simulink model "platoon_project_string_stability2"  (Simulink 8.9)
settings: Solver=VariableStepAuto  StartTime=0.0  StopTime=20  FixedStep=0.1  RelTol=1e-3  EnableMultiTasking=on
values from neighbouring files (symbols this model uses):
  k1 = 1.3244    [platoon_stability.m]    (also in platoon_stability_ed.m = 0.0244)
  k2 = -1.2211    [platoon_stability.m]    (also in platoon_stability_ed.m = -1.7211)
  q = 0.1    [platoon_stability.m]    (also in platoon_stability_ed.m = 0.2)
  tau = 1.34    [platoon_stability.m]    (also in platoon_stability_ed.m = 1.24)
  tnet_table = [57.5127074443 119.897368421 182.282029398 223.675296349 261.549751738 274.206057597 279.305263158 283.689473684 288.073684211 292.467532318 296.875779086 301.284025854 ... (400 elements, 20x20)]    [enginemap.mat]    (also in genmap.m = griddata(map_ford(:,1), map_ford(:,4), map_ford(:,2), we_tab)
  we_max = 471.2    [enginemap.mat]    (also in genmap.m = max(map_ford(:,1)))
  we_min = 57.6    [enginemap.mat]    (also in genmap.m = min(map_ford(:,1)))
undefined symbols (not defined in the file or in its folder): c_aero, delay_brake, F_roll, h, I_e, I_wheel, KB, mass, max_throttle, max_throttle_rate, min_throttle, mu_B, mu_C, mu_D, mu_E, P_po, Rdrive, sigbuilder_block, tau_brake, tau_throttle, throttle_o, w_wheel_o, we_o, x_dot_o
libraries: simulink x8
(part 2 of 3)

== system platoon_project_string_stability2/4th Vehicle/Engine Model ==
  note: engine map이 저장되어있다
      | 2-D Lookup table
      |
      | input : Throttle angle, Engine speed
      | output : Engine torque
  Tractive Force : Inport
  Throttle Angle : Inport  Port=2
  Brake Torque : Inport  Port=3
  Gear Ratio : Inport  Port=4
  1/(I_e+4*I_w*R^2) : Fcn  Expr=u(1)/(I_e+4*I_wheel*u(2)^2)
  Integrator : Integrator  InitialCondition=we_o  LimitOutput=on  UpperSaturationLimit=[we_max]  LowerSaturationLimit=[we_min]
  Mux : Mux  Inputs=2
  Product : Product  SaturateOnIntegerOverflow=on  RndMeth=Zero  InputSameDT=on  OutDataTypeStr=Inherit: Same as first input
  Sum : Sum  Inputs=+|-  SaturateOnIntegerOverflow=on  InputSameDT=on  OutDataTypeStr=Inherit: Same as first input
  Sum1 : Sum  SaturateOnIntegerOverflow=on  InputSameDT=on  OutDataTypeStr=Inherit: Same as first input
  T_net : Lookup2D  RowIndex=alpha_table  ColumnIndex=we_table  Table=tnet_table  SaturateOnIntegerOverflow=on  InputSameDT=on
  wheel radius : Gain  Gain=h  Multiplication=Matrix(K*u)  SaturateOnIntegerOverflow=on  OutDataTypeStr=Inherit: Same as input  ParamDataTypeStr=Inherit: Same as input
  Engine Speed : Outport
  Engine Torque : Outport  Port=2
  wires:
  Throttle Angle/1 -> T_net/1
  Integrator/1 -> Engine Speed/1, T_net/2  "w"
  1/(I_e+4*I_w*R^2)/1 -> Integrator/1  "w_dot"
  Tractive Force/1 -> wheel radius/1
  wheel radius/1 -> Sum1/1
  Brake Torque/1 -> Sum1/2
  Product/1 -> Sum/2
  Sum1/1 -> Product/1
  Gear Ratio/1 -> Product/2, Mux/2
  Sum/1 -> Mux/1
  Mux/1 -> 1/(I_e+4*I_w*R^2)/1
  T_net/1 -> Engine Torque/1, Sum/1

== system platoon_project_string_stability2/4th Vehicle/Gear Shift ==
  note: [1 1 1]인 [n,1] 행렬과
      | 반환행렬을 곱해서
      | 스칼라값(기어값)을 만든다
  note: 현재 차량 속도 vs 기어변속 속도를 비교한다
      | [0; 1; 1] 같은 [1,n]행렬이 반환된다
  Vehicle Speed : Inport
  Convert m/s to mph : Gain  Gain=3.6/1.6  SaturateOnIntegerOverflow=on  OutDataTypeStr=Inherit: Same as input  ParamDataTypeStr=Inherit: Same as input
  Direct Look-Up of Gear ratio : LookupNDDirect  NumberOfTableDimensions=1  Table=[0.3423,0.6378,1.0,1.4184]
  Get gear-1 : Gain  Gain=ones(1,3)  Multiplication=Matrix(K*u)  SaturateOnIntegerOverflow=on  OutDataTypeStr=Inherit: Same as input  ParamDataTypeStr=Inherit: Same as input
  Relational Operator : RelationalOperator  Operator=>  RndMeth=Nearest  InputSameDT=on
  Shift Speeds : Constant  Value=[15 32 67]
  Gear Ratio : Outport
  wires:
  Shift Speeds/1 -> Relational Operator/2
  Relational Operator/1 -> Get gear-1/1
  Convert m/s to mph/1 -> Relational Operator/1
  Get gear-1/1 -> Direct Look-Up of Gear ratio/1
  Vehicle Speed/1 -> Convert m/s to mph/1
  Direct Look-Up of Gear ratio/1 -> Gear Ratio/1

== system platoon_project_string_stability2/4th Vehicle/Throttle Actuator ==
  Command : Inport
  Integrator : Integrator  InitialCondition=throttle_o  LimitOutput=on  UpperSaturationLimit=max_throttle  LowerSaturationLimit=min_throttle
  Saturation : Saturate  UpperLimit=max_throttle_rate  LowerLimit=-max_throttle_rate
  Sum : Sum  Inputs=-+|  SaturateOnIntegerOverflow=on  InputSameDT=on  OutDataTypeStr=Inherit: Same as first input
  Throttle Time Constant : Gain  Gain=1/tau_throttle  SaturateOnIntegerOverflow=on  OutDataTypeStr=Inherit: Same as input  ParamDataTypeStr=Inherit: Same as input
  Angle : Outport
  wires:
  Command/1 -> Sum/2
  Integrator/1 -> Angle/1, Sum/1
  Sum/1 -> Throttle Time Constant/1
  Throttle Time Constant/1 -> Saturation/1
  Saturation/1 -> Integrator/1

== system platoon_project_string_stability2/4th Vehicle/Vehicle Dynamics ==
  note: 타이어저항 F_road
  note: v
  note: v_dot
  note: 공기저항 F_air
  note: 구름저항 F_roll
  note: Initial Velocity = 21 [m/s]
  Tractive Force : Inport
  Aerodynamic Drag : Fcn  Expr=c_aero*u^2
  Divide by Mass : Gain  Gain=1/mass  Multiplication=Matrix(K*u)  SaturateOnIntegerOverflow=on  OutDataTypeStr=Inherit: Same as input  ParamDataTypeStr=Inherit: Same as input
  Integrator : Integrator  InitialCondition=x_dot_o  LimitOutput=on  LowerSaturationLimit=0
  Rolling Resistance : Constant  Value=F_roll
  Sum1 : Sum  Inputs=--+  SaturateOnIntegerOverflow=on  InputSameDT=on  OutDataTypeStr=Inherit: Same as first input
  Velocity : Outport
  Acceleration : Outport  Port=2
  wires:
  Tractive Force/1 -> Sum1/3
  Divide by Mass/1 -> Acceleration/1, Integrator/1
  Integrator/1 -> Velocity/1, Aerodynamic Drag/1
  Sum1/1 -> Divide by Mass/1
  Rolling Resistance/1 -> Sum1/2
  Aerodynamic Drag/1 -> Sum1/1

== system platoon_project_string_stability2/4th Vehicle/Wheel Dynamics ==
  note: 여기 주석!
  note: Tractive Force는 4바퀴 전부 더한다
  note: 평균을 계산해서 하나의 Wheel Speed를 만든다
  note: 브레이크는 전체 유압을
      | 전륜, 후륜에 특정비율로 분배한다
      | 40% (전륜), 60% (후륜)
  Vehicle Speed : Inport
  T_shaft : Inport  Port=2
  Brake Torque : Inport  Port=3
  Average Speed : Gain  Gain=0.25*ones(1,4)  Multiplication=Matrix(K*u)  SaturateOnIntegerOverflow=on  OutDataTypeStr=Inherit: Same as input  ParamDataTypeStr=Inherit: Same as input
  Front Brake Distribution : Gain  Gain=0.2  SaturateOnIntegerOverflow=on  OutDataTypeStr=Inherit: Same as input  ParamDataTypeStr=Inherit: Same as input
  Front Wheel Drive : Gain  Gain=0.5  SaturateOnIntegerOverflow=on  OutDataTypeStr=Inherit: Same as input  ParamDataTypeStr=Inherit: Same as input
  Left Front Wheel : Subsystem
  Left Rear Wheel : Subsystem
  Mux : Mux
  Mux1 : Mux
  Mux2 : Mux
  Rear Brake Distribution : Gain  Gain=0.3  SaturateOnIntegerOverflow=on  OutDataTypeStr=Inherit: Same as input  ParamDataTypeStr=Inherit: Same as input
  Right Front Wheel : Subsystem
  Right Rear Wheel : Subsystem
  Terminator : Terminator
  Total Tractive Force : Gain  Gain=ones(1,4)  Multiplication=Matrix(K*u)  SaturateOnIntegerOverflow=on  OutDataTypeStr=Inherit: Same as input  ParamDataTypeStr=Inherit: Same as input
  Wheel Speeds : Scope
  Tractive Force : Outport
  Wheel Speed : Outport  Port=2
  wires:
  Total Tractive Force/1 -> Tractive Force/1
  Average Speed/1 -> Wheel Speed/1
  Mux/1 -> Total Tractive Force/1
  Vehicle Speed/1 -> Right Front Wheel/2(Vehicle Speed), Left Rear Wheel/3(Vehicle Speed), Right Rear Wheel/3(Vehicle Speed), Left Front Wheel/2(Vehicle Speed)
  Right Front Wheel/1(Tractive Force) -> Mux/1
  Left Front Wheel/1(Tractive Force) -> Mux/2
  Right Rear Wheel/1(Tractive Force) -> Mux/3
  Left Rear Wheel/1(Tractive Force) -> Mux/4
  Mux1/1 -> Average Speed/1, Wheel Speeds/1
  Right Front Wheel/2(Wheel Speed) -> Mux1/1
  Left Front Wheel/2(Wheel Speed) -> Mux1/2
  Right Rear Wheel/2(Wheel Speed) -> Mux1/3
  Left Rear Wheel/2(Wheel Speed) -> Mux1/4
  Right Front Wheel/3(RF_slip) -> Mux2/1
  Left Rear Wheel/3(LR_slip) -> Mux2/4
  Mux2/1 -> Terminator/1
  T_shaft/1 -> Front Wheel Drive/1
  Front Wheel Drive/1 -> Right Rear Wheel/1(T_shaft), Left Rear Wheel/1(T_shaft)
  Brake Torque/1 -> Rear Brake Distribution/1, Front Brake Distribution/1
  Left Front Wheel/3(LF_slip) -> Mux2/2
  Right Rear Wheel/3(RR_slip) -> Mux2/3
  Front Brake Distribution/1 -> Right Front Wheel/1(T_brake), Left Front Wheel/1(T_brake)
  Rear Brake Distribution/1 -> Left Rear Wheel/2(T_brake), Right Rear Wheel/2(T_brake)

== system platoon_project_string_stability2/1st Vehicle/Wheel Dynamics/Left Front Wheel ==
  T_brake : Inport
  Vehicle Speed : Inport  Port=2
  1/inertia : Gain  Gain=1/I_wheel  SaturateOnIntegerOverflow=on  OutDataTypeStr=Inherit: Same as input  ParamDataTypeStr=Inherit: Same as input
  Integrator : Integrator  InitialCondition=w_wheel_o
  Sum : Sum  Inputs=-|-  SaturateOnIntegerOverflow=on  InputSameDT=on  OutDataTypeStr=Inherit: Same as first input
  Tire Model : Subsystem
  wheel radius : Gain  Gain=h  SaturateOnIntegerOverflow=on  OutDataTypeStr=Inherit: Same as input  ParamDataTypeStr=Inherit: Same as input
  Tractive Force : Outport
  Wheel Speed : Outport  Port=2
  LF_slip : Outport  Port=3
  wires:
  Tire Model/2(LF_slip) -> LF_slip/1
  Tire Model/1(Tractive Force) -> wheel radius/1, Tractive Force/1
  Vehicle Speed/1 -> Tire Model/2(Vehicle Speed)
  wheel radius/1 -> Sum/2
  T_brake/1 -> Sum/1
  Integrator/1 -> Tire Model/1(Wheel Speed), Wheel Speed/1
  Sum/1 -> 1/inertia/1
  1/inertia/1 -> Integrator/1

== system platoon_project_string_stability2/1st Vehicle/Wheel Dynamics/Left Rear Wheel ==
  note: w_dot
  note: w
  note: T_shaft
  note: T_brake
  note: h*F_road
  note: Wheel Dynamics
  T_shaft : Inport
  T_brake : Inport  Port=2
  Vehicle Speed : Inport  Port=3
  1/inertia : Gain  Gain=1/I_wheel  SaturateOnIntegerOverflow=on  OutDataTypeStr=Inherit: Same as input  ParamDataTypeStr=Inherit: Same as input
  Integrator : Integrator  InitialCondition=w_wheel_o
  Sum : Sum  Inputs=+--  SaturateOnIntegerOverflow=on  InputSameDT=on  OutDataTypeStr=Inherit: Same as first input
  Tire Model : Subsystem
  wheel radius : Gain  Gain=h  SaturateOnIntegerOverflow=on  OutDataTypeStr=Inherit: Same as input  ParamDataTypeStr=Inherit: Same as input
  Tractive Force : Outport
  Wheel Speed : Outport  Port=2
  LR_slip : Outport  Port=3
  wires:
  wheel radius/1 -> Sum/3
  T_brake/1 -> Sum/2
  T_shaft/1 -> Sum/1
  Tire Model/2(LR_slip) -> LR_slip/1
  Tire Model/1(Tractive Force) -> wheel radius/1, Tractive Force/1
  Vehicle Speed/1 -> Tire Model/2(Vehicle Speed)
  Integrator/1 -> Tire Model/1(Wheel Speed), Wheel Speed/1
  Sum/1 -> 1/inertia/1
  1/inertia/1 -> Integrator/1

== system platoon_project_string_stability2/1st Vehicle/Wheel Dynamics/Right Front Wheel ==
  note: w_dot
  note: w
  T_brake : Inport
  Vehicle Speed : Inport  Port=2
  1/inertia : Gain  Gain=1/I_wheel  SaturateOnIntegerOverflow=on  OutDataTypeStr=Inherit: Same as input  ParamDataTypeStr=Inherit: Same as input
  Integrator : Integrator  InitialCondition=w_wheel_o
  Sum : Sum  Inputs=|--  SaturateOnIntegerOverflow=on  InputSameDT=on  OutDataTypeStr=Inherit: Same as first input
  Tire Model : Subsystem
  wheel radius : Gain  Gain=h  SaturateOnIntegerOverflow=on  OutDataTypeStr=Inherit: Same as input  ParamDataTypeStr=Inherit: Same as input
  Tractive Force : Outport
  Wheel Speed : Outport  Port=2
  RF_slip : Outport  Port=3
  wires:
  T_brake/1 -> Sum/1
  wheel radius/1 -> Sum/2
  Tire Model/2(RF_slip) -> RF_slip/1
  Tire Model/1(Tractive Force) -> wheel radius/1, Tractive Force/1
  Vehicle Speed/1 -> Tire Model/2(Vehicle Speed)
  Integrator/1 -> Tire Model/1(Wheel Speed), Wheel Speed/1
  Sum/1 -> 1/inertia/1
  1/inertia/1 -> Integrator/1

== system platoon_project_string_stability2/1st Vehicle/Wheel Dynamics/Right Rear Wheel ==
  T_shaft : Inport
  T_brake : Inport  Port=2
  Vehicle Speed : Inport  Port=3
  1/inertia : Gain  Gain=1/I_wheel  SaturateOnIntegerOverflow=on  OutDataTypeStr=Inherit: Same as input  ParamDataTypeStr=Inherit: Same as input
  Integrator : Integrator  InitialCondition=w_wheel_o
  Sum : Sum  Inputs=+--  SaturateOnIntegerOverflow=on  InputSameDT=on  OutDataTypeStr=Inherit: Same as first input
  Tire Model : Subsystem
  wheel radius : Gain  Gain=h  SaturateOnIntegerOverflow=on  OutDataTypeStr=Inherit: Same as input  ParamDataTypeStr=Inherit: Same as input
  Tractive Force : Outport
  Wheel Speed : Outport  Port=2
  RR_slip : Outport  Port=3
  wires:
  T_shaft/1 -> Sum/1
  wheel radius/1 -> Sum/3
  T_brake/1 -> Sum/2
  Tire Model/2(RR_slip) -> RR_slip/1
  Tire Model/1(Tractive Force) -> wheel radius/1, Tractive Force/1
  Vehicle Speed/1 -> Tire Model/2(Vehicle Speed)
  Integrator/1 -> Tire Model/1(Wheel Speed), Wheel Speed/1
  Sum/1 -> 1/inertia/1
  1/inertia/1 -> Integrator/1

== system platoon_project_string_stability2/2nd Vehicle/Wheel Dynamics/Left Front Wheel ==
  T_brake : Inport
  Vehicle Speed : Inport  Port=2
  1/inertia : Gain  Gain=1/I_wheel  SaturateOnIntegerOverflow=on  OutDataTypeStr=Inherit: Same as input  ParamDataTypeStr=Inherit: Same as input
  Integrator : Integrator  InitialCondition=w_wheel_o
  Sum : Sum  Inputs=-|-  SaturateOnIntegerOverflow=on  InputSameDT=on  OutDataTypeStr=Inherit: Same as first input
  Tire Model : Subsystem
  wheel radius : Gain  Gain=h  SaturateOnIntegerOverflow=on  OutDataTypeStr=Inherit: Same as input  ParamDataTypeStr=Inherit: Same as input
  Tractive Force : Outport
  Wheel Speed : Outport  Port=2
  LF_slip : Outport  Port=3
  wires:
  1/inertia/1 -> Integrator/1
  Sum/1 -> 1/inertia/1
  Integrator/1 -> Wheel Speed/1, Tire Model/1(Wheel Speed)
  T_brake/1 -> Sum/1
  wheel radius/1 -> Sum/2
  Vehicle Speed/1 -> Tire Model/2(Vehicle Speed)
  Tire Model/1(Tractive Force) -> Tractive Force/1, wheel radius/1
  Tire Model/2(LF_slip) -> LF_slip/1

== system platoon_project_string_stability2/2nd Vehicle/Wheel Dynamics/Left Rear Wheel ==
  note: Wheel Dynamics
  note: h*F_road
  note: T_brake
  note: T_shaft
  note: w
  note: w_dot
  T_shaft : Inport
  T_brake : Inport  Port=2
  Vehicle Speed : Inport  Port=3
  1/inertia : Gain  Gain=1/I_wheel  SaturateOnIntegerOverflow=on  OutDataTypeStr=Inherit: Same as input  ParamDataTypeStr=Inherit: Same as input
  Integrator : Integrator  InitialCondition=w_wheel_o
  Sum : Sum  Inputs=+--  SaturateOnIntegerOverflow=on  InputSameDT=on  OutDataTypeStr=Inherit: Same as first input
  Tire Model : Subsystem
  wheel radius : Gain  Gain=h  SaturateOnIntegerOverflow=on  OutDataTypeStr=Inherit: Same as input  ParamDataTypeStr=Inherit: Same as input
  Tractive Force : Outport
  Wheel Speed : Outport  Port=2
  LR_slip : Outport  Port=3
  wires:
  1/inertia/1 -> Integrator/1
  Sum/1 -> 1/inertia/1
  Integrator/1 -> Wheel Speed/1, Tire Model/1(Wheel Speed)
  Vehicle Speed/1 -> Tire Model/2(Vehicle Speed)
  Tire Model/1(Tractive Force) -> Tractive Force/1, wheel radius/1
  Tire Model/2(LR_slip) -> LR_slip/1
  T_shaft/1 -> Sum/1
  T_brake/1 -> Sum/2
  wheel radius/1 -> Sum/3

== system platoon_project_string_stability2/2nd Vehicle/Wheel Dynamics/Right Front Wheel ==
  note: w
  note: w_dot
  T_brake : Inport
  Vehicle Speed : Inport  Port=2
  1/inertia : Gain  Gain=1/I_wheel  SaturateOnIntegerOverflow=on  OutDataTypeStr=Inherit: Same as input  ParamDataTypeStr=Inherit: Same as input
  Integrator : Integrator  InitialCondition=w_wheel_o
  Sum : Sum  Inputs=|--  SaturateOnIntegerOverflow=on  InputSameDT=on  OutDataTypeStr=Inherit: Same as first input
  Tire Model : Subsystem
  wheel radius : Gain  Gain=h  SaturateOnIntegerOverflow=on  OutDataTypeStr=Inherit: Same as input  ParamDataTypeStr=Inherit: Same as input
  Tractive Force : Outport
  Wheel Speed : Outport  Port=2
  RF_slip : Outport  Port=3
  wires:
  1/inertia/1 -> Integrator/1
  Sum/1 -> 1/inertia/1
  Integrator/1 -> Wheel Speed/1, Tire Model/1(Wheel Speed)
  Vehicle Speed/1 -> Tire Model/2(Vehicle Speed)
  Tire Model/1(Tractive Force) -> Tractive Force/1, wheel radius/1
  Tire Model/2(RF_slip) -> RF_slip/1
  wheel radius/1 -> Sum/2
  T_brake/1 -> Sum/1

== system platoon_project_string_stability2/2nd Vehicle/Wheel Dynamics/Right Rear Wheel ==
  T_shaft : Inport
  T_brake : Inport  Port=2
  Vehicle Speed : Inport  Port=3
  1/inertia : Gain  Gain=1/I_wheel  SaturateOnIntegerOverflow=on  OutDataTypeStr=Inherit: Same as input  ParamDataTypeStr=Inherit: Same as input
  Integrator : Integrator  InitialCondition=w_wheel_o
  Sum : Sum  Inputs=+--  SaturateOnIntegerOverflow=on  InputSameDT=on  OutDataTypeStr=Inherit: Same as first input
  Tire Model : Subsystem
  wheel radius : Gain  Gain=h  SaturateOnIntegerOverflow=on  OutDataTypeStr=Inherit: Same as input  ParamDataTypeStr=Inherit: Same as input
  Tractive Force : Outport
  Wheel Speed : Outport  Port=2
  RR_slip : Outport  Port=3
  wires:
  1/inertia/1 -> Integrator/1
  Sum/1 -> 1/inertia/1
  Integrator/1 -> Wheel Speed/1, Tire Model/1(Wheel Speed)
  Vehicle Speed/1 -> Tire Model/2(Vehicle Speed)
  Tire Model/1(Tractive Force) -> Tractive Force/1, wheel radius/1
  Tire Model/2(RR_slip) -> RR_slip/1
  T_brake/1 -> Sum/2
  wheel radius/1 -> Sum/3
  T_shaft/1 -> Sum/1

== system platoon_project_string_stability2/3rd Vehicle/Wheel Dynamics/Left Front Wheel ==
  T_brake : Inport
  Vehicle Speed : Inport  Port=2
  1/inertia : Gain  Gain=1/I_wheel  SaturateOnIntegerOverflow=on  OutDataTypeStr=Inherit: Same as input  ParamDataTypeStr=Inherit: Same as input
  Integrator : Integrator  InitialCondition=w_wheel_o
  Sum : Sum  Inputs=-|-  SaturateOnIntegerOverflow=on  InputSameDT=on  OutDataTypeStr=Inherit: Same as first input
  Tire Model : Subsystem
  wheel radius : Gain  Gain=h  SaturateOnIntegerOverflow=on  OutDataTypeStr=Inherit: Same as input  ParamDataTypeStr=Inherit: Same as input
  Tractive Force : Outport
  Wheel Speed : Outport  Port=2
  LF_slip : Outport  Port=3
  wires:
  Tire Model/2(LF_slip) -> LF_slip/1
  Tire Model/1(Tractive Force) -> wheel radius/1, Tractive Force/1
  Vehicle Speed/1 -> Tire Model/2(Vehicle Speed)
  wheel radius/1 -> Sum/2
  T_brake/1 -> Sum/1
  Integrator/1 -> Tire Model/1(Wheel Speed), Wheel Speed/1
  Sum/1 -> 1/inertia/1
  1/inertia/1 -> Integrator/1

== system platoon_project_string_stability2/3rd Vehicle/Wheel Dynamics/Left Rear Wheel ==
  note: w_dot
  note: w
  note: T_shaft
  note: T_brake
  note: h*F_road
  note: Wheel Dynamics
  T_shaft : Inport
  T_brake : Inport  Port=2
  Vehicle Speed : Inport  Port=3
  1/inertia : Gain  Gain=1/I_wheel  SaturateOnIntegerOverflow=on  OutDataTypeStr=Inherit: Same as input  ParamDataTypeStr=Inherit: Same as input
  Integrator : Integrator  InitialCondition=w_wheel_o
  Sum : Sum  Inputs=+--  SaturateOnIntegerOverflow=on  InputSameDT=on  OutDataTypeStr=Inherit: Same as first input
  Tire Model : Subsystem
  wheel radius : Gain  Gain=h  SaturateOnIntegerOverflow=on  OutDataTypeStr=Inherit: Same as input  ParamDataTypeStr=Inherit: Same as input
  Tractive Force : Outport
  Wheel Speed : Outport  Port=2
  LR_slip : Outport  Port=3
  wires:
  wheel radius/1 -> Sum/3
  T_brake/1 -> Sum/2
  T_shaft/1 -> Sum/1
  Tire Model/2(LR_slip) -> LR_slip/1
  Tire Model/1(Tractive Force) -> wheel radius/1, Tractive Force/1
  Vehicle Speed/1 -> Tire Model/2(Vehicle Speed)
  Integrator/1 -> Tire Model/1(Wheel Speed), Wheel Speed/1
  Sum/1 -> 1/inertia/1
  1/inertia/1 -> Integrator/1

== system platoon_project_string_stability2/3rd Vehicle/Wheel Dynamics/Right Front Wheel ==
  note: w_dot
  note: w
  T_brake : Inport
  Vehicle Speed : Inport  Port=2
  1/inertia : Gain  Gain=1/I_wheel  SaturateOnIntegerOverflow=on  OutDataTypeStr=Inherit: Same as input  ParamDataTypeStr=Inherit: Same as input
  Integrator : Integrator  InitialCondition=w_wheel_o
  Sum : Sum  Inputs=|--  SaturateOnIntegerOverflow=on  InputSameDT=on  OutDataTypeStr=Inherit: Same as first input
  Tire Model : Subsystem
  wheel radius : Gain  Gain=h  SaturateOnIntegerOverflow=on  OutDataTypeStr=Inherit: Same as input  ParamDataTypeStr=Inherit: Same as input
  Tractive Force : Outport
  Wheel Speed : Outport  Port=2
  RF_slip : Outport  Port=3
  wires:
  T_brake/1 -> Sum/1
  wheel radius/1 -> Sum/2
  Tire Model/2(RF_slip) -> RF_slip/1
  Tire Model/1(Tractive Force) -> wheel radius/1, Tractive Force/1
  Vehicle Speed/1 -> Tire Model/2(Vehicle Speed)
  Integrator/1 -> Tire Model/1(Wheel Speed), Wheel Speed/1
  Sum/1 -> 1/inertia/1
  1/inertia/1 -> Integrator/1

== system platoon_project_string_stability2/3rd Vehicle/Wheel Dynamics/Right Rear Wheel ==
  T_shaft : Inport
  T_brake : Inport  Port=2
  Vehicle Speed : Inport  Port=3
  1/inertia : Gain  Gain=1/I_wheel  SaturateOnIntegerOverflow=on  OutDataTypeStr=Inherit: Same as input  ParamDataTypeStr=Inherit: Same as input
  Integrator : Integrator  InitialCondition=w_wheel_o
  Sum : Sum  Inputs=+--  SaturateOnIntegerOverflow=on  InputSameDT=on  OutDataTypeStr=Inherit: Same as first input
  Tire Model : Subsystem
  wheel radius : Gain  Gain=h  SaturateOnIntegerOverflow=on  OutDataTypeStr=Inherit: Same as input  ParamDataTypeStr=Inherit: Same as input
  Tractive Force : Outport
  Wheel Speed : Outport  Port=2
  RR_slip : Outport  Port=3
  wires:
  T_shaft/1 -> Sum/1
  wheel radius/1 -> Sum/3
  T_brake/1 -> Sum/2
  Tire Model/2(RR_slip) -> RR_slip/1
  Tire Model/1(Tractive Force) -> wheel radius/1, Tractive Force/1
  Vehicle Speed/1 -> Tire Model/2(Vehicle Speed)
  Integrator/1 -> Tire Model/1(Wheel Speed), Wheel Speed/1
  Sum/1 -> 1/inertia/1
  1/inertia/1 -> Integrator/1

== system platoon_project_string_stability2/4th Vehicle/Wheel Dynamics/Left Front Wheel ==
  T_brake : Inport
  Vehicle Speed : Inport  Port=2
  1/inertia : Gain  Gain=1/I_wheel  SaturateOnIntegerOverflow=on  OutDataTypeStr=Inherit: Same as input  ParamDataTypeStr=Inherit: Same as input
  Integrator : Integrator  InitialCondition=w_wheel_o
  Sum : Sum  Inputs=-|-  SaturateOnIntegerOverflow=on  InputSameDT=on  OutDataTypeStr=Inherit: Same as first input
  Tire Model : Subsystem
  wheel radius : Gain  Gain=h  SaturateOnIntegerOverflow=on  OutDataTypeStr=Inherit: Same as input  ParamDataTypeStr=Inherit: Same as input
  Tractive Force : Outport
  Wheel Speed : Outport  Port=2
  LF_slip : Outport  Port=3
  wires:
  1/inertia/1 -> Integrator/1
  Sum/1 -> 1/inertia/1
  Integrator/1 -> Wheel Speed/1, Tire Model/1(Wheel Speed)
  T_brake/1 -> Sum/1
  wheel radius/1 -> Sum/2
  Vehicle Speed/1 -> Tire Model/2(Vehicle Speed)
  Tire Model/1(Tractive Force) -> Tractive Force/1, wheel radius/1
  Tire Model/2(LF_slip) -> LF_slip/1

== system platoon_project_string_stability2/4th Vehicle/Wheel Dynamics/Left Rear Wheel ==
  note: Wheel Dynamics
  note: h*F_road
  note: T_brake
  note: T_shaft
  note: w
  note: w_dot
  T_shaft : Inport
  T_brake : Inport  Port=2
  Vehicle Speed : Inport  Port=3
  1/inertia : Gain  Gain=1/I_wheel  SaturateOnIntegerOverflow=on  OutDataTypeStr=Inherit: Same as input  ParamDataTypeStr=Inherit: Same as input
  Integrator : Integrator  InitialCondition=w_wheel_o
  Sum : Sum  Inputs=+--  SaturateOnIntegerOverflow=on  InputSameDT=on  OutDataTypeStr=Inherit: Same as first input
  Tire Model : Subsystem
  wheel radius : Gain  Gain=h  SaturateOnIntegerOverflow=on  OutDataTypeStr=Inherit: Same as input  ParamDataTypeStr=Inherit: Same as input
  Tractive Force : Outport
  Wheel Speed : Outport  Port=2
  LR_slip : Outport  Port=3
  wires:
  1/inertia/1 -> Integrator/1
  Sum/1 -> 1/inertia/1
  Integrator/1 -> Wheel Speed/1, Tire Model/1(Wheel Speed)
  Vehicle Speed/1 -> Tire Model/2(Vehicle Speed)
  Tire Model/1(Tractive Force) -> Tractive Force/1, wheel radius/1
  Tire Model/2(LR_slip) -> LR_slip/1
  T_shaft/1 -> Sum/1
  T_brake/1 -> Sum/2
  wheel radius/1 -> Sum/3

== system platoon_project_string_stability2/4th Vehicle/Wheel Dynamics/Right Front Wheel ==
  note: w
  note: w_dot
  T_brake : Inport
  Vehicle Speed : Inport  Port=2
  1/inertia : Gain  Gain=1/I_wheel  SaturateOnIntegerOverflow=on  OutDataTypeStr=Inherit: Same as input  ParamDataTypeStr=Inherit: Same as input
  Integrator : Integrator  InitialCondition=w_wheel_o
  Sum : Sum  Inputs=|--  SaturateOnIntegerOverflow=on  InputSameDT=on  OutDataTypeStr=Inherit: Same as first input
  Tire Model : Subsystem
  wheel radius : Gain  Gain=h  SaturateOnIntegerOverflow=on  OutDataTypeStr=Inherit: Same as input  ParamDataTypeStr=Inherit: Same as input
  Tractive Force : Outport
  Wheel Speed : Outport  Port=2
  RF_slip : Outport  Port=3
  wires:
  1/inertia/1 -> Integrator/1
  Sum/1 -> 1/inertia/1
  Integrator/1 -> Wheel Speed/1, Tire Model/1(Wheel Speed)
  Vehicle Speed/1 -> Tire Model/2(Vehicle Speed)
  Tire Model/1(Tractive Force) -> Tractive Force/1, wheel radius/1
  Tire Model/2(RF_slip) -> RF_slip/1
  wheel radius/1 -> Sum/2
  T_brake/1 -> Sum/1

== system platoon_project_string_stability2/4th Vehicle/Wheel Dynamics/Right Rear Wheel ==
  T_shaft : Inport
  T_brake : Inport  Port=2
  Vehicle Speed : Inport  Port=3
  1/inertia : Gain  Gain=1/I_wheel  SaturateOnIntegerOverflow=on  OutDataTypeStr=Inherit: Same as input  ParamDataTypeStr=Inherit: Same as input
  Integrator : Integrator  InitialCondition=w_wheel_o
  Sum : Sum  Inputs=+--  SaturateOnIntegerOverflow=on  InputSameDT=on  OutDataTypeStr=Inherit: Same as first input
  Tire Model : Subsystem
  wheel radius : Gain  Gain=h  SaturateOnIntegerOverflow=on  OutDataTypeStr=Inherit: Same as input  ParamDataTypeStr=Inherit: Same as input
  Tractive Force : Outport
  Wheel Speed : Outport  Port=2
  RR_slip : Outport  Port=3
  wires:
  1/inertia/1 -> Integrator/1
  Sum/1 -> 1/inertia/1
  Integrator/1 -> Wheel Speed/1, Tire Model/1(Wheel Speed)
  Vehicle Speed/1 -> Tire Model/2(Vehicle Speed)
  Tire Model/1(Tractive Force) -> Tractive Force/1, wheel radius/1
  Tire Model/2(RR_slip) -> RR_slip/1
  T_brake/1 -> Sum/2
  wheel radius/1 -> Sum/3
  T_shaft/1 -> Sum/1

== system platoon_project_string_stability2/1st Vehicle/Wheel Dynamics/Left Front Wheel/Tire Model ==
  Wheel Speed : Inport
  Vehicle Speed : Inport  Port=2
  Constant : Constant  Value=0.01
  Constant1 : Constant  Value=0.01
  Fcn : Fcn  Expr=mu_D*sin(mu_C*atan(mu_B*u-mu_E*(mu_B*u-atan(mu_B*u))))
  Gain : Gain  SaturateOnIntegerOverflow=on  OutDataTypeStr=Inherit: Same as input  ParamDataTypeStr=Inherit: Same as input
  Product : Product  Inputs=/*  SaturateOnIntegerOverflow=on  RndMeth=Zero  InputSameDT=on  OutDataTypeStr=Inherit: Same as first input
  Product1 : Product  Inputs=*/  SaturateOnIntegerOverflow=on  RndMeth=Zero  InputSameDT=on  OutDataTypeStr=Inherit: Same as first input
  Sum1 : Sum  Inputs=+-  SaturateOnIntegerOverflow=on  InputSameDT=on  OutDataTypeStr=Inherit: Same as first input
  Switch : Switch  SaturateOnIntegerOverflow=on  InputSameDT=on
  Switch1 : Switch  Threshold=0.01  SaturateOnIntegerOverflow=on  InputSameDT=on
  Switch2 : Switch  Threshold=0.01  SaturateOnIntegerOverflow=on  InputSameDT=on
  wheel radius1 : Gain  Gain=h  SaturateOnIntegerOverflow=on  OutDataTypeStr=Inherit: Same as input  ParamDataTypeStr=Inherit: Same as input
  Tractive Force : Outport
  LF_slip : Outport  Port=2
  wires:
  Constant1/1 -> Switch2/3
  Switch2/1 -> Product1/2
  Switch1/1 -> Product/1
  Constant/1 -> Switch1/3
  Gain/1 -> Fcn/1
  Vehicle Speed/1 -> Switch2/2, Switch2/1, Sum1/2
  Fcn/1 -> Tractive Force/1
  Wheel Speed/1 -> wheel radius1/1
  Switch/1 -> LF_slip/1, Gain/1  "slip"
  Product1/1 -> Switch/3
  Product/1 -> Switch/1
  Sum1/1 -> Product1/1, Product/2, Switch/2
  wheel radius1/1 -> Switch1/2, Switch1/1, Sum1/1

== system platoon_project_string_stability2/1st Vehicle/Wheel Dynamics/Left Rear Wheel/Tire Model ==
  note: divide by 0를 없애기 위해
      | Switch Block을 사용했다
  note: Slip ratio
  note: rw-v
  note: Magic Tire Formula
  Wheel Speed : Inport
  Vehicle Speed : Inport  Port=2
  Constant : Constant  Value=0.01
  Constant1 : Constant  Value=0.01
  Fcn : Fcn  Expr=mu_D*sin(mu_C*atan(mu_B*u-mu_E*(mu_B*u-atan(mu_B*u))))
  Gain : Gain  SaturateOnIntegerOverflow=on  OutDataTypeStr=Inherit: Same as input  ParamDataTypeStr=Inherit: Same as input
  Product : Product  Inputs=/*  SaturateOnIntegerOverflow=on  RndMeth=Zero  InputSameDT=on  OutDataTypeStr=Inherit: Same as first input
  Product1 : Product  Inputs=*/  SaturateOnIntegerOverflow=on  RndMeth=Zero  InputSameDT=on  OutDataTypeStr=Inherit: Same as first input
  Sum1 : Sum  Inputs=+-  SaturateOnIntegerOverflow=on  InputSameDT=on  OutDataTypeStr=Inherit: Same as first input
  Switch : Switch  SaturateOnIntegerOverflow=on  InputSameDT=on
  Switch1 : Switch  Threshold=0.01  SaturateOnIntegerOverflow=on  InputSameDT=on
  Switch2 : Switch  Threshold=0.01  SaturateOnIntegerOverflow=on  InputSameDT=on
  wheel radius1 : Gain  Gain=h  SaturateOnIntegerOverflow=on  OutDataTypeStr=Inherit: Same as input  ParamDataTypeStr=Inherit: Same as input
  Tractive Force : Outport
  LR_slip : Outport  Port=2
  wires:
  Constant1/1 -> Switch2/3
  Switch2/1 -> Product1/2
  Switch1/1 -> Product/1
  Constant/1 -> Switch1/3
  Gain/1 -> Fcn/1
  Vehicle Speed/1 -> Switch2/2, Switch2/1, Sum1/2
  Fcn/1 -> Tractive Force/1
  Wheel Speed/1 -> wheel radius1/1
  Switch/1 -> LR_slip/1, Gain/1  "slip"
  Product1/1 -> Switch/3
  Product/1 -> Switch/1
  Sum1/1 -> Product1/1, Product/2, Switch/2
  wheel radius1/1 -> Switch1/2, Switch1/1, Sum1/1

== system platoon_project_string_stability2/1st Vehicle/Wheel Dynamics/Right Front Wheel/Tire Model ==
  note: divide by 0를 없애기 위해
      | Switch Block을 사용했다
  note: Slip ratio
  note: Magic Tire Formula
  note: rw-v
  Wheel Speed : Inport
  Vehicle Speed : Inport  Port=2
  Constant : Constant  Value=0.01
  Constant1 : Constant  Value=0.01
  Fcn : Fcn  Expr=mu_D*sin(mu_C*atan(mu_B*u-mu_E*(mu_B*u-atan(mu_B*u))))
  Gain : Gain  SaturateOnIntegerOverflow=on  OutDataTypeStr=Inherit: Same as input  ParamDataTypeStr=Inherit: Same as input
  Product : Product  Inputs=/*  SaturateOnIntegerOverflow=on  RndMeth=Zero  InputSameDT=on  OutDataTypeStr=Inherit: Same as first input
  Product1 : Product  Inputs=*/  SaturateOnIntegerOverflow=on  RndMeth=Zero  InputSameDT=on  OutDataTypeStr=Inherit: Same as first input
  Sum1 : Sum  Inputs=+-  SaturateOnIntegerOverflow=on  InputSameDT=on  OutDataTypeStr=Inherit: Same as first input
  Switch : Switch  SaturateOnIntegerOverflow=on  InputSameDT=on
  Switch1 : Switch  Threshold=0.01  SaturateOnIntegerOverflow=on  InputSameDT=on
  Switch2 : Switch  Threshold=0.01  SaturateOnIntegerOverflow=on  InputSameDT=on
  wheel radius1 : Gain  Gain=h  SaturateOnIntegerOverflow=on  OutDataTypeStr=Inherit: Same as input  ParamDataTypeStr=Inherit: Same as input
  Tractive Force : Outport
  RF_slip : Outport  Port=2
  wires:
  Constant1/1 -> Switch2/3
  Switch2/1 -> Product1/2
  Switch1/1 -> Product/1
  Constant/1 -> Switch1/3
  Gain/1 -> Fcn/1
  Vehicle Speed/1 -> Switch2/2, Switch2/1, Sum1/2
  Fcn/1 -> Tractive Force/1
  Wheel Speed/1 -> wheel radius1/1
  Switch/1 -> RF_slip/1, Gain/1  "slip"
  Product1/1 -> Switch/3
  Product/1 -> Switch/1
  Sum1/1 -> Product1/1, Product/2, Switch/2
  wheel radius1/1 -> Switch1/2, Switch1/1, Sum1/1

== system platoon_project_string_stability2/1st Vehicle/Wheel Dynamics/Right Rear Wheel/Tire Model ==
  Wheel Speed : Inport
  Vehicle Speed : Inport  Port=2
  Constant : Constant  Value=0.01
  Constant1 : Constant  Value=0.01
  Fcn : Fcn  Expr=mu_D*sin(mu_C*atan(mu_B*u-mu_E*(mu_B*u-atan(mu_B*u))))
  Gain : Gain  SaturateOnIntegerOverflow=on  OutDataTypeStr=Inherit: Same as input  ParamDataTypeStr=Inherit: Same as input
  Product : Product  Inputs=/*  SaturateOnIntegerOverflow=on  RndMeth=Zero  InputSameDT=on  OutDataTypeStr=Inherit: Same as first input
  Product1 : Product  Inputs=*/  SaturateOnIntegerOverflow=on  RndMeth=Zero  InputSameDT=on  OutDataTypeStr=Inherit: Same as first input
  Sum1 : Sum  Inputs=+-  SaturateOnIntegerOverflow=on  InputSameDT=on  OutDataTypeStr=Inherit: Same as first input
  Switch : Switch  SaturateOnIntegerOverflow=on  InputSameDT=on
  Switch1 : Switch  Threshold=0.01  SaturateOnIntegerOverflow=on  InputSameDT=on
  Switch2 : Switch  Threshold=0.01  SaturateOnIntegerOverflow=on  InputSameDT=on
  wheel radius1 : Gain  Gain=h  SaturateOnIntegerOverflow=on  OutDataTypeStr=Inherit: Same as input  ParamDataTypeStr=Inherit: Same as input
  Tractive Force : Outport
  RR_slip : Outport  Port=2
  wires:
  Constant1/1 -> Switch2/3
  Switch2/1 -> Product1/2
  Switch1/1 -> Product/1
  Constant/1 -> Switch1/3
  Gain/1 -> Fcn/1
  Vehicle Speed/1 -> Switch2/2, Switch2/1, Sum1/2
  Fcn/1 -> Tractive Force/1
  Wheel Speed/1 -> wheel radius1/1
  Switch/1 -> RR_slip/1, Gain/1  "slip"
  Product1/1 -> Switch/3
  Product/1 -> Switch/1
  Sum1/1 -> Product1/1, Product/2, Switch/2
  wheel radius1/1 -> Switch1/2, Switch1/1, Sum1/1

== system platoon_project_string_stability2/2nd Vehicle/Wheel Dynamics/Left Front Wheel/Tire Model ==
  Wheel Speed : Inport
  Vehicle Speed : Inport  Port=2
  Constant : Constant  Value=0.01
  Constant1 : Constant  Value=0.01
  Fcn : Fcn  Expr=mu_D*sin(mu_C*atan(mu_B*u-mu_E*(mu_B*u-atan(mu_B*u))))
  Gain : Gain  SaturateOnIntegerOverflow=on  OutDataTypeStr=Inherit: Same as input  ParamDataTypeStr=Inherit: Same as input
  Product : Product  Inputs=/*  SaturateOnIntegerOverflow=on  RndMeth=Zero  InputSameDT=on  OutDataTypeStr=Inherit: Same as first input
  Product1 : Product  Inputs=*/  SaturateOnIntegerOverflow=on  RndMeth=Zero  InputSameDT=on  OutDataTypeStr=Inherit: Same as first input
  Sum1 : Sum  Inputs=+-  SaturateOnIntegerOverflow=on  InputSameDT=on  OutDataTypeStr=Inherit: Same as first input
  Switch : Switch  SaturateOnIntegerOverflow=on  InputSameDT=on
  Switch1 : Switch  Threshold=0.01  SaturateOnIntegerOverflow=on  InputSameDT=on
  Switch2 : Switch  Threshold=0.01  SaturateOnIntegerOverflow=on  InputSameDT=on
  wheel radius1 : Gain  Gain=h  SaturateOnIntegerOverflow=on  OutDataTypeStr=Inherit: Same as input  ParamDataTypeStr=Inherit: Same as input
  Tractive Force : Outport
  LF_slip : Outport  Port=2
  wires:
  wheel radius1/1 -> Sum1/1, Switch1/1, Switch1/2
  Sum1/1 -> Switch/2, Product/2, Product1/1
  Product/1 -> Switch/1
  Product1/1 -> Switch/3
  Switch/1 -> Gain/1, LF_slip/1  "slip"
  Wheel Speed/1 -> wheel radius1/1
  Fcn/1 -> Tractive Force/1
  Vehicle Speed/1 -> Sum1/2, Switch2/1, Switch2/2
  Gain/1 -> Fcn/1
  Constant/1 -> Switch1/3
  Switch1/1 -> Product/1
  Switch2/1 -> Product1/2
  Constant1/1 -> Switch2/3

== system platoon_project_string_stability2/2nd Vehicle/Wheel Dynamics/Left Rear Wheel/Tire Model ==
  note: Magic Tire Formula
  note: rw-v
  note: Slip ratio
  note: divide by 0를 없애기 위해
      | Switch Block을 사용했다
  Wheel Speed : Inport
  Vehicle Speed : Inport  Port=2
  Constant : Constant  Value=0.01
  Constant1 : Constant  Value=0.01
  Fcn : Fcn  Expr=mu_D*sin(mu_C*atan(mu_B*u-mu_E*(mu_B*u-atan(mu_B*u))))
  Gain : Gain  SaturateOnIntegerOverflow=on  OutDataTypeStr=Inherit: Same as input  ParamDataTypeStr=Inherit: Same as input
  Product : Product  Inputs=/*  SaturateOnIntegerOverflow=on  RndMeth=Zero  InputSameDT=on  OutDataTypeStr=Inherit: Same as first input
  Product1 : Product  Inputs=*/  SaturateOnIntegerOverflow=on  RndMeth=Zero  InputSameDT=on  OutDataTypeStr=Inherit: Same as first input
  Sum1 : Sum  Inputs=+-  SaturateOnIntegerOverflow=on  InputSameDT=on  OutDataTypeStr=Inherit: Same as first input
  Switch : Switch  SaturateOnIntegerOverflow=on  InputSameDT=on
  Switch1 : Switch  Threshold=0.01  SaturateOnIntegerOverflow=on  InputSameDT=on
  Switch2 : Switch  Threshold=0.01  SaturateOnIntegerOverflow=on  InputSameDT=on
  wheel radius1 : Gain  Gain=h  SaturateOnIntegerOverflow=on  OutDataTypeStr=Inherit: Same as input  ParamDataTypeStr=Inherit: Same as input
  Tractive Force : Outport
  LR_slip : Outport  Port=2
  wires:
  wheel radius1/1 -> Sum1/1, Switch1/1, Switch1/2
  Sum1/1 -> Switch/2, Product/2, Product1/1
  Product/1 -> Switch/1
  Product1/1 -> Switch/3
  Switch/1 -> Gain/1, LR_slip/1  "slip"
  Wheel Speed/1 -> wheel radius1/1
  Fcn/1 -> Tractive Force/1
  Vehicle Speed/1 -> Sum1/2, Switch2/1, Switch2/2
  Gain/1 -> Fcn/1
  Constant/1 -> Switch1/3
  Switch1/1 -> Product/1
  Switch2/1 -> Product1/2
  Constant1/1 -> Switch2/3

== system platoon_project_string_stability2/2nd Vehicle/Wheel Dynamics/Right Front Wheel/Tire Model ==
  note: rw-v
  note: Magic Tire Formula
  note: Slip ratio
  note: divide by 0를 없애기 위해
      | Switch Block을 사용했다
  Wheel Speed : Inport
  Vehicle Speed : Inport  Port=2
  Constant : Constant  Value=0.01
  Constant1 : Constant  Value=0.01
  Fcn : Fcn  Expr=mu_D*sin(mu_C*atan(mu_B*u-mu_E*(mu_B*u-atan(mu_B*u))))
  Gain : Gain  SaturateOnIntegerOverflow=on  OutDataTypeStr=Inherit: Same as input  ParamDataTypeStr=Inherit: Same as input
  Product : Product  Inputs=/*  SaturateOnIntegerOverflow=on  RndMeth=Zero  InputSameDT=on  OutDataTypeStr=Inherit: Same as first input
  Product1 : Product  Inputs=*/  SaturateOnIntegerOverflow=on  RndMeth=Zero  InputSameDT=on  OutDataTypeStr=Inherit: Same as first input
  Sum1 : Sum  Inputs=+-  SaturateOnIntegerOverflow=on  InputSameDT=on  OutDataTypeStr=Inherit: Same as first input
  Switch : Switch  SaturateOnIntegerOverflow=on  InputSameDT=on
  Switch1 : Switch  Threshold=0.01  SaturateOnIntegerOverflow=on  InputSameDT=on
  Switch2 : Switch  Threshold=0.01  SaturateOnIntegerOverflow=on  InputSameDT=on
  wheel radius1 : Gain  Gain=h  SaturateOnIntegerOverflow=on  OutDataTypeStr=Inherit: Same as input  ParamDataTypeStr=Inherit: Same as input
  Tractive Force : Outport
  RF_slip : Outport  Port=2
  wires:
  wheel radius1/1 -> Sum1/1, Switch1/1, Switch1/2
  Sum1/1 -> Switch/2, Product/2, Product1/1
  Product/1 -> Switch/1
  Product1/1 -> Switch/3
  Switch/1 -> Gain/1, RF_slip/1  "slip"
  Wheel Speed/1 -> wheel radius1/1
  Fcn/1 -> Tractive Force/1
  Vehicle Speed/1 -> Sum1/2, Switch2/1, Switch2/2
  Gain/1 -> Fcn/1
  Constant/1 -> Switch1/3
  Switch1/1 -> Product/1
  Switch2/1 -> Product1/2
  Constant1/1 -> Switch2/3

== system platoon_project_string_stability2/2nd Vehicle/Wheel Dynamics/Right Rear Wheel/Tire Model ==
  Wheel Speed : Inport
  Vehicle Speed : Inport  Port=2
  Constant : Constant  Value=0.01
  Constant1 : Constant  Value=0.01
  Fcn : Fcn  Expr=mu_D*sin(mu_C*atan(mu_B*u-mu_E*(mu_B*u-atan(mu_B*u))))
  Gain : Gain  SaturateOnIntegerOverflow=on  OutDataTypeStr=Inherit: Same as input  ParamDataTypeStr=Inherit: Same as input
  Product : Product  Inputs=/*  SaturateOnIntegerOverflow=on  RndMeth=Zero  InputSameDT=on  OutDataTypeStr=Inherit: Same as first input
  Product1 : Product  Inputs=*/  SaturateOnIntegerOverflow=on  RndMeth=Zero  InputSameDT=on  OutDataTypeStr=Inherit: Same as first input
  Sum1 : Sum  Inputs=+-  SaturateOnIntegerOverflow=on  InputSameDT=on  OutDataTypeStr=Inherit: Same as first input
  Switch : Switch  SaturateOnIntegerOverflow=on  InputSameDT=on
  Switch1 : Switch  Threshold=0.01  SaturateOnIntegerOverflow=on  InputSameDT=on
  Switch2 : Switch  Threshold=0.01  SaturateOnIntegerOverflow=on  InputSameDT=on
  wheel radius1 : Gain  Gain=h  SaturateOnIntegerOverflow=on  OutDataTypeStr=Inherit: Same as input  ParamDataTypeStr=Inherit: Same as input
  Tractive Force : Outport
  RR_slip : Outport  Port=2
  wires:
  wheel radius1/1 -> Sum1/1, Switch1/1, Switch1/2
  Sum1/1 -> Switch/2, Product/2, Product1/1
  Product/1 -> Switch/1
  Product1/1 -> Switch/3
  Switch/1 -> Gain/1, RR_slip/1  "slip"
  Wheel Speed/1 -> wheel radius1/1
  Fcn/1 -> Tractive Force/1
  Vehicle Speed/1 -> Sum1/2, Switch2/1, Switch2/2
  Gain/1 -> Fcn/1
  Constant/1 -> Switch1/3
  Switch1/1 -> Product/1
  Switch2/1 -> Product1/2
  Constant1/1 -> Switch2/3

== system platoon_project_string_stability2/3rd Vehicle/Wheel Dynamics/Left Front Wheel/Tire Model ==
  Wheel Speed : Inport
  Vehicle Speed : Inport  Port=2
  Constant : Constant  Value=0.01
  Constant1 : Constant  Value=0.01
  Fcn : Fcn  Expr=mu_D*sin(mu_C*atan(mu_B*u-mu_E*(mu_B*u-atan(mu_B*u))))
  Gain : Gain  SaturateOnIntegerOverflow=on  OutDataTypeStr=Inherit: Same as input  ParamDataTypeStr=Inherit: Same as input
  Product : Product  Inputs=/*  SaturateOnIntegerOverflow=on  RndMeth=Zero  InputSameDT=on  OutDataTypeStr=Inherit: Same as first input
  Product1 : Product  Inputs=*/  SaturateOnIntegerOverflow=on  RndMeth=Zero  InputSameDT=on  OutDataTypeStr=Inherit: Same as first input
  Sum1 : Sum  Inputs=+-  SaturateOnIntegerOverflow=on  InputSameDT=on  OutDataTypeStr=Inherit: Same as first input
  Switch : Switch  SaturateOnIntegerOverflow=on  InputSameDT=on
  Switch1 : Switch  Threshold=0.01  SaturateOnIntegerOverflow=on  InputSameDT=on
  Switch2 : Switch  Threshold=0.01  SaturateOnIntegerOverflow=on  InputSameDT=on
  wheel radius1 : Gain  Gain=h  SaturateOnIntegerOverflow=on  OutDataTypeStr=Inherit: Same as input  ParamDataTypeStr=Inherit: Same as input
  Tractive Force : Outport
  LF_slip : Outport  Port=2
  wires:
  Constant1/1 -> Switch2/3
  Switch2/1 -> Product1/2
  Switch1/1 -> Product/1
  Constant/1 -> Switch1/3
  Gain/1 -> Fcn/1
  Vehicle Speed/1 -> Switch2/2, Switch2/1, Sum1/2
  Fcn/1 -> Tractive Force/1
  Wheel Speed/1 -> wheel radius1/1
  Switch/1 -> LF_slip/1, Gain/1  "slip"
  Product1/1 -> Switch/3
  Product/1 -> Switch/1
  Sum1/1 -> Product1/1, Product/2, Switch/2
  wheel radius1/1 -> Switch1/2, Switch1/1, Sum1/1

== system platoon_project_string_stability2/3rd Vehicle/Wheel Dynamics/Left Rear Wheel/Tire Model ==
  note: divide by 0를 없애기 위해
      | Switch Block을 사용했다
  note: Slip ratio
  note: rw-v
  note: Magic Tire Formula
  Wheel Speed : Inport
  Vehicle Speed : Inport  Port=2
  Constant : Constant  Value=0.01
  Constant1 : Constant  Value=0.01
  Fcn : Fcn  Expr=mu_D*sin(mu_C*atan(mu_B*u-mu_E*(mu_B*u-atan(mu_B*u))))
  Gain : Gain  SaturateOnIntegerOverflow=on  OutDataTypeStr=Inherit: Same as input  ParamDataTypeStr=Inherit: Same as input
  Product : Product  Inputs=/*  SaturateOnIntegerOverflow=on  RndMeth=Zero  InputSameDT=on  OutDataTypeStr=Inherit: Same as first input
  Product1 : Product  Inputs=*/  SaturateOnIntegerOverflow=on  RndMeth=Zero  InputSameDT=on  OutDataTypeStr=Inherit: Same as first input
  Sum1 : Sum  Inputs=+-  SaturateOnIntegerOverflow=on  InputSameDT=on  OutDataTypeStr=Inherit: Same as first input
  Switch : Switch  SaturateOnIntegerOverflow=on  InputSameDT=on
  Switch1 : Switch  Threshold=0.01  SaturateOnIntegerOverflow=on  InputSameDT=on
  Switch2 : Switch  Threshold=0.01  SaturateOnIntegerOverflow=on  InputSameDT=on
  wheel radius1 : Gain  Gain=h  SaturateOnIntegerOverflow=on  OutDataTypeStr=Inherit: Same as input  ParamDataTypeStr=Inherit: Same as input
  Tractive Force : Outport
  LR_slip : Outport  Port=2
  wires:
  Constant1/1 -> Switch2/3
  Switch2/1 -> Product1/2
  Switch1/1 -> Product/1
  Constant/1 -> Switch1/3
  Gain/1 -> Fcn/1
  Vehicle Speed/1 -> Switch2/2, Switch2/1, Sum1/2
  Fcn/1 -> Tractive Force/1
  Wheel Speed/1 -> wheel radius1/1
  Switch/1 -> LR_slip/1, Gain/1  "slip"
  Product1/1 -> Switch/3
  Product/1 -> Switch/1
  Sum1/1 -> Product1/1, Product/2, Switch/2
  wheel radius1/1 -> Switch1/2, Switch1/1, Sum1/1

== system platoon_project_string_stability2/3rd Vehicle/Wheel Dynamics/Right Front Wheel/Tire Model ==
  note: divide by 0를 없애기 위해
      | Switch Block을 사용했다
  note: Slip ratio
  note: Magic Tire Formula
  note: rw-v
  Wheel Speed : Inport
  Vehicle Speed : Inport  Port=2
  Constant : Constant  Value=0.01
  Constant1 : Constant  Value=0.01
  Fcn : Fcn  Expr=mu_D*sin(mu_C*atan(mu_B*u-mu_E*(mu_B*u-atan(mu_B*u))))
  Gain : Gain  SaturateOnIntegerOverflow=on  OutDataTypeStr=Inherit: Same as input  ParamDataTypeStr=Inherit: Same as input
  Product : Product  Inputs=/*  SaturateOnIntegerOverflow=on  RndMeth=Zero  InputSameDT=on  OutDataTypeStr=Inherit: Same as first input
  Product1 : Product  Inputs=*/  SaturateOnIntegerOverflow=on  RndMeth=Zero  InputSameDT=on  OutDataTypeStr=Inherit: Same as first input
  Sum1 : Sum  Inputs=+-  SaturateOnIntegerOverflow=on  InputSameDT=on  OutDataTypeStr=Inherit: Same as first input
  Switch : Switch  SaturateOnIntegerOverflow=on  InputSameDT=on
  Switch1 : Switch  Threshold=0.01  SaturateOnIntegerOverflow=on  InputSameDT=on
  Switch2 : Switch  Threshold=0.01  SaturateOnIntegerOverflow=on  InputSameDT=on
  wheel radius1 : Gain  Gain=h  SaturateOnIntegerOverflow=on  OutDataTypeStr=Inherit: Same as input  ParamDataTypeStr=Inherit: Same as input
  Tractive Force : Outport
  RF_slip : Outport  Port=2
  wires:
  Constant1/1 -> Switch2/3
  Switch2/1 -> Product1/2
  Switch1/1 -> Product/1
  Constant/1 -> Switch1/3
  Gain/1 -> Fcn/1
  Vehicle Speed/1 -> Switch2/2, Switch2/1, Sum1/2
  Fcn/1 -> Tractive Force/1
  Wheel Speed/1 -> wheel radius1/1
  Switch/1 -> RF_slip/1, Gain/1  "slip"
  Product1/1 -> Switch/3
  Product/1 -> Switch/1
  Sum1/1 -> Product1/1, Product/2, Switch/2
  wheel radius1/1 -> Switch1/2, Switch1/1, Sum1/1

== system platoon_project_string_stability2/3rd Vehicle/Wheel Dynamics/Right Rear Wheel/Tire Model ==
  Wheel Speed : Inport
  Vehicle Speed : Inport  Port=2
  Constant : Constant  Value=0.01
  Constant1 : Constant  Value=0.01
  Fcn : Fcn  Expr=mu_D*sin(mu_C*atan(mu_B*u-mu_E*(mu_B*u-atan(mu_B*u))))
  Gain : Gain  SaturateOnIntegerOverflow=on  OutDataTypeStr=Inherit: Same as input  ParamDataTypeStr=Inherit: Same as input
  Product : Product  Inputs=/*  SaturateOnIntegerOverflow=on  RndMeth=Zero  InputSameDT=on  OutDataTypeStr=Inherit: Same as first input
  Product1 : Product  Inputs=*/  SaturateOnIntegerOverflow=on  RndMeth=Zero  InputSameDT=on  OutDataTypeStr=Inherit: Same as first input
  Sum1 : Sum  Inputs=+-  SaturateOnIntegerOverflow=on  InputSameDT=on  OutDataTypeStr=Inherit: Same as first input
  Switch : Switch  SaturateOnIntegerOverflow=on  InputSameDT=on
  Switch1 : Switch  Threshold=0.01  SaturateOnIntegerOverflow=on  InputSameDT=on
  Switch2 : Switch  Threshold=0.01  SaturateOnIntegerOverflow=on  InputSameDT=on
  wheel radius1 : Gain  Gain=h  SaturateOnIntegerOverflow=on  OutDataTypeStr=Inherit: Same as input  ParamDataTypeStr=Inherit: Same as input
  Tractive Force : Outport
  RR_slip : Outport  Port=2
  wires:
  Constant1/1 -> Switch2/3
  Switch2/1 -> Product1/2
  Switch1/1 -> Product/1
  Constant/1 -> Switch1/3
  Gain/1 -> Fcn/1
  Vehicle Speed/1 -> Switch2/2, Switch2/1, Sum1/2
  Fcn/1 -> Tractive Force/1
  Wheel Speed/1 -> wheel radius1/1
  Switch/1 -> RR_slip/1, Gain/1  "slip"
  Product1/1 -> Switch/3
  Product/1 -> Switch/1
  Sum1/1 -> Product1/1, Product/2, Switch/2
  wheel radius1/1 -> Switch1/2, Switch1/1, Sum1/1

== system platoon_project_string_stability2/4th Vehicle/Wheel Dynamics/Left Front Wheel/Tire Model ==
  Wheel Speed : Inport
  Vehicle Speed : Inport  Port=2
  Constant : Constant  Value=0.01
  Constant1 : Constant  Value=0.01
  Fcn : Fcn  Expr=mu_D*sin(mu_C*atan(mu_B*u-mu_E*(mu_B*u-atan(mu_B*u))))
  Gain : Gain  SaturateOnIntegerOverflow=on  OutDataTypeStr=Inherit: Same as input  ParamDataTypeStr=Inherit: Same as input
  Product : Product  Inputs=/*  SaturateOnIntegerOverflow=on  RndMeth=Zero  InputSameDT=on  OutDataTypeStr=Inherit: Same as first input
  Product1 : Product  Inputs=*/  SaturateOnIntegerOverflow=on  RndMeth=Zero  InputSameDT=on  OutDataTypeStr=Inherit: Same as first input
  Sum1 : Sum  Inputs=+-  SaturateOnIntegerOverflow=on  InputSameDT=on  OutDataTypeStr=Inherit: Same as first input
  Switch : Switch  SaturateOnIntegerOverflow=on  InputSameDT=on
  Switch1 : Switch  Threshold=0.01  SaturateOnIntegerOverflow=on  InputSameDT=on
  Switch2 : Switch  Threshold=0.01  SaturateOnIntegerOverflow=on  InputSameDT=on
  wheel radius1 : Gain  Gain=h  SaturateOnIntegerOverflow=on  OutDataTypeStr=Inherit: Same as input  ParamDataTypeStr=Inherit: Same as input
  Tractive Force : Outport
  LF_slip : Outport  Port=2
  wires:
  wheel radius1/1 -> Sum1/1, Switch1/1, Switch1/2
  Sum1/1 -> Switch/2, Product/2, Product1/1
  Product/1 -> Switch/1
  Product1/1 -> Switch/3
  Switch/1 -> Gain/1, LF_slip/1  "slip"
  Wheel Speed/1 -> wheel radius1/1
  Fcn/1 -> Tractive Force/1
  Vehicle Speed/1 -> Sum1/2, Switch2/1, Switch2/2
  Gain/1 -> Fcn/1
  Constant/1 -> Switch1/3
  Switch1/1 -> Product/1
  Switch2/1 -> Product1/2
  Constant1/1 -> Switch2/3

== system platoon_project_string_stability2/4th Vehicle/Wheel Dynamics/Left Rear Wheel/Tire Model ==
  note: Magic Tire Formula
  note: rw-v
  note: Slip ratio
  note: divide by 0를 없애기 위해
      | Switch Block을 사용했다
  Wheel Speed : Inport
  Vehicle Speed : Inport  Port=2
  Constant : Constant  Value=0.01
  Constant1 : Constant  Value=0.01
  Fcn : Fcn  Expr=mu_D*sin(mu_C*atan(mu_B*u-mu_E*(mu_B*u-atan(mu_B*u))))
  Gain : Gain  SaturateOnIntegerOverflow=on  OutDataTypeStr=Inherit: Same as input  ParamDataTypeStr=Inherit: Same as input
  Product : Product  Inputs=/*  SaturateOnIntegerOverflow=on  RndMeth=Zero  InputSameDT=on  OutDataTypeStr=Inherit: Same as first input
  Product1 : Product  Inputs=*/  SaturateOnIntegerOverflow=on  RndMeth=Zero  InputSameDT=on  OutDataTypeStr=Inherit: Same as first input
  Sum1 : Sum  Inputs=+-  SaturateOnIntegerOverflow=on  InputSameDT=on  OutDataTypeStr=Inherit: Same as first input
  Switch : Switch  SaturateOnIntegerOverflow=on  InputSameDT=on
  Switch1 : Switch  Threshold=0.01  SaturateOnIntegerOverflow=on  InputSameDT=on
  Switch2 : Switch  Threshold=0.01  SaturateOnIntegerOverflow=on  InputSameDT=on
  wheel radius1 : Gain  Gain=h  SaturateOnIntegerOverflow=on  OutDataTypeStr=Inherit: Same as input  ParamDataTypeStr=Inherit: Same as input
  Tractive Force : Outport
  LR_slip : Outport  Port=2
  wires:
  wheel radius1/1 -> Sum1/1, Switch1/1, Switch1/2
  Sum1/1 -> Switch/2, Product/2, Product1/1
  Product/1 -> Switch/1
  Product1/1 -> Switch/3
  Switch/1 -> Gain/1, LR_slip/1  "slip"
  Wheel Speed/1 -> wheel radius1/1
  Fcn/1 -> Tractive Force/1
  Vehicle Speed/1 -> Sum1/2, Switch2/1, Switch2/2
  Gain/1 -> Fcn/1
  Constant/1 -> Switch1/3
  Switch1/1 -> Product/1
  Switch2/1 -> Product1/2
  Constant1/1 -> Switch2/3
